simulink model "CAR_CONTROL_SYSTEM"  (R2024b)
settings: Solver=FixedStepAuto  StartTime=0.0  StopTime=inf  FixedStep=1e-3  RelTol=1e-3  EnableMultiTasking=on
model workspace (MAT data in the model file):
  SL_ROS_VariableLengthArrays_MaxSizes : object (value not decoded)
undefined symbols (not defined in the file or in its folder): angular, CIRCUIT, CLTF_DAMP, CLTF_FREQ, CLTF_GAIN, CONTROL, CONTROL_INI, DiscIntNeverNeededParam, dspblkCoreblockFVToolHelper, gcbh, INPUT, linear, MCP3201, MD25, MODEL, MODEL_INI, mpcstate, MPU60X0, MPU9250, MSG, NAV_MPC_CONTROL, OUTPUT, SAMPLING_TIME, SYSID_INPUT, VL6180X
libraries: raspberrypiCommlib x153, simulink x85, raspberrypiNetworklib x8, embedlinuxBasiclib x6, ctrlSharedLib x2, ros2lib x2, mpclib x1, vrlib x1, sldrtlib x1
(part 14 of 16)

== matlab function CAR_CONTROL_SYSTEM/SIMULATION/CAR MODEL  ==
  settings: updateMethod=DISCRETE  sampleTime=MODEL_INI.PARAM.SIM_SAMPLING_TIME
  data: STATE input; MODEL_IN input; STATE_DERIVATIVE output; MODEL output Bus: MODEL_Bus
function [STATE_DERIVATIVE,MODEL] = CAR_MODEL(STATE,MODEL_IN)
%% COPY MODEL_BUS
MODEL = MODEL_IN;

%% Reference frames
% Fixed or earth reference frame
% X,e1I - North
% Y,e2I - East
% Z,e3I - Down
% Body reference frame with origin in the center of mass
% Xb,e1B - forward axis
% Yb,e2B - right axis
% Zb,e3B - downward axis

persistent initialize TIMER
if isempty(initialize)
    TIMER = 0;
    initialize = 1;
end

%--------------------------------------------------------------
% MOTOR PARAMETERS
%--------------------------------------------------------------
% Rotor resistance (ohm)
Rm = MODEL.PARAM.MOTOR_RESISTANCE;
% Motor back-emf constant (V/rad*s)
Ke = MODEL.PARAM.MOTOR_BEMF_CONSTANT;
% Torque constant (N.m/A)
Kt = MODEL.PARAM.MOTOR_TORQUE_CONSTANT;
% Motor static torque (N. m) eje motor
Trmax = MODEL.PARAM.MOTOR_STATIC_TORQUE; 
% Viscous friction coefficient in the motor axis (N.m.s/rad)
Dm = MODEL.PARAM.MOTOR_VISCOUS_FRICTION_COEFF;
% Motor + wheel inertia in the motor axis (kg.m^2)
Im = MODEL.PARAM.MOTOR_INERTIA;
% Motor gear ratio
n1 = MODEL.PARAM.MOTOR_GEAR_RATIO;
% Converter voltage drop (V)
vc_drop = MODEL.PARAM.MOTOR_VOLT_DROP_COM;
vd_drop = MODEL.PARAM.MOTOR_VOLT_DROP_DIF;

%--------------------------------------------------------------
% CAR PARAMETERS
%--------------------------------------------------------------
% Body mass without wheels (kg)
M = MODEL.PARAM.BODY_MASS; 
% Wheel mass including the rotor (kg)
m = MODEL.PARAM.WHEEL_MASS;
% Body inertia in x-axis (kg.m^2)
Ix = MODEL.PARAM.BODY_INERTIA_X;
% Body inertia in y-axis (pitch) (kg.m^2)
Iy = MODEL.PARAM.BODY_INERTIA_Y;
% Body inertia in z-axis (kg.m^2)
Iz = MODEL.PARAM.BODY_INERTIA_Z;
% Viscous friction coefficient in x-axis (N.m.s/rad)
Dx = MODEL.PARAM.BODY_VISCOUS_FRICTION_COEFF_X;
% Viscous friction coefficient in z-axis (N.m.s/rad)
Dz = MODEL.PARAM.BODY_VISCOUS_FRICTION_COEFF_Z;
% Center of gravity distance from the wheel axis (m)
h = MODEL.PARAM.BODY_DISTANCE;
% Wheel radius (m)
R = MODEL.PARAM.WHEEL_RADIUS;
% Distance between wheels (m)
W = MODEL.PARAM.WHEEL_DISTANCE;
% Wheel gear ratio 
n2 = MODEL.PARAM.WHEEL_GEAR_RATIO; 

%--------------------------------------------------------------
% OTHER PARAMETERS
%--------------------------------------------------------------
% Gravity (m/s^2)
g = MODEL.PARAM.GRAVITY;
% Vehicle mode: / 0. CAR / 1. SELF-BALANCING VEHICLE
vmode = MODEL.PARAM.VEHICLE_MODE;
% Yaw and range sensor parameters
if vmode == 0 % CAR
    Iyaw = Iz;
    Dyaw = Dz;
    if MODEL.PARAM.WALL_FOLLOWER_MODE
        xA = MODEL.PARAM.LIDAR_2D_XA;
        yA = MODEL.PARAM.LIDAR_2D_YA;        
    else
        xA = MODEL.PARAM.RANGE_XA;
        yA = MODEL.PARAM.RANGE_YA;
    end
else % SELF-BALANCING VEHICLE
    Iyaw = Ix;
    Dyaw = Dx;
    xA = MODEL.PARAM.RANGE_ZA;
    yA = MODEL.PARAM.RANGE_YA;  
end

%--------------------------------------------------------------
% STATE VARIABLES
%--------------------------------------------------------------
% Forward velocity (m/s)
vc = STATE(1);
% Yaw rate
dShi = STATE(2);
% Yaw angle
Shi = STATE(3);
% Position in earth x-axis (m)
x = STATE(4);
% Position in earth y-axis (m)
y = STATE(5);
% Wall follower mode
if (MODEL.PARAM.CONTROL_MODE == 4) || (MODEL.PARAM.CONTROL_MODE == 5)
    % Wall distance (m)
    d_wall = STATE(6);
    % Wall angle (rad)
    Shi_wall = STATE(7);
else
    d_wall = 0;
    Shi_wall = 0;
end
% Pitch rate (rad/s)
dTheta = STATE(8);
% Pitch angle (rad)
Theta = STATE(9);
if abs(Theta)>=pi/2
    dTheta = 0;
end

%--------------------------------------------------------------
% INPUT VARIABLES
%--------------------------------------------------------------
% Motor voltages (V)
ul = MODEL.INPUT.MOTOR_VOLT(1);
ur = MODEL.INPUT.MOTOR_VOLT(2);
% Wall rotation (rad/s)
w_wall = MODEL.INPUT.WALL_RATE;

%%%%%%%%%%%%%%%%%%%%%%%%%%%%%%%%%%%%%%%%%%%%%%%%%%%%%%%%%%%%%%%%%%%%%%%%%%%
% STATE EQUATIONS
%%%%%%%%%%%%%%%%%%%%%%%%%%%%%%%%%%%%%%%%%%%%%%%%%%%%%%%%%%%%%%%%%%%%%%%%%%%
%--------------------------------------------------------------
% Common  motor voltage (V)
uc = (ul+ur)/2;
% Differential motor voltage (V)
ud = (ul-ur)/2;
%--------------------------------------------------------------
% Differential velocity of the wheels (m/s)
vd = W/2*dShi;
% (wml-wmr)/2/n2*R/W
% Common angular rate of the wheels (rad/s)
wc = vc/R;
% Differential angular rate of the wheels (rad/s)
wd = vd/R;
%--------------------------------------------------------------
% Common angular rate of the motors (rad/s)
wmc = n2*wc + dTheta/n1;
% Differential angular rate of the motors (rad/s)
wmd = n2*wd;
%--------------------------------------------------------------
% Motor rate 
wml = wmc + wmd;
wmr = wmc - wmd;
% wmc = (wmr+wml)/2;
% wmd = (wml-wmr)/2
%--------------------------------------------------------------
% Motor equations
el = Ke*wml;
er = Ke*wmr;
vl_drop = sign(ul-el)*(vc_drop+vd_drop);
vr_drop = sign(ur-er)*(vc_drop-vd_drop);
if abs(ul-el)<vl_drop
    vl_drop = 0;    
end
if abs(ur-er)<vr_drop
    vr_drop = 0;
end
% Currents
il = (ul-vl_drop-el)/Rm;
ir = (ur-vr_drop-er)/Rm;
% ic = (il+ir)/2;
% id = (il-ir)/2;
% dil = (ul - el - Rm*il)/Lm;
% dir = (ur - er - Rm*ir)/Lm;
% Motor torques
Tml = Kt*il;
Tmr = Kt*ir;
Tmc = (Tml+Tmr)/2;
Tmd = (Tml-Tmr)/2;
%--------------------------------------------------------------
% Static friction torques
Trl_lim = Tml*(abs(Tml)<Trmax) - Trmax*(Tml<=-Trmax) + Trmax*(Tml>=Trmax);
Trl = Trl_lim*(abs(wml)==0) + Trmax*sign(wml)*(abs(wml)>0);
Trr_lim = Tmr*(abs(Tmr)<Trmax) - Trmax*(Tmr<=-Trmax) + Trmax*(Tmr>=Trmax);
Trr = Trr_lim*(abs(wmr)==0) + Trmax*sign(wmr)*(abs(wmr)>0);
Trc = (Trl+Trr)/2;
Trd = (Trl-Trr)/2;
%--------------------------------------------------------------
% Viscous friction torques
Tdl = Dm*wml;
Tdr = Dm*wmr;
Tdc = (Tdr+Tdl)/2;
Tdd = (Tdl-Tdr)/2;
%--------------------------------------------------------------
% Total motor torque
% Tl = Tml - Tdl - Trl - Frl*R/n2;
% Tr = Tmr - Tdr - Trr - Frr*R/n2;
%--------------------------------------------------------------
% Motor angular accelerations
% dwml = Tl/Im = (Tml-Tdl-Trl-Frl*R/n2)/Im
% dwmr = Tr/Im = (Tmr-Tdr-Trr-Frr*R/n2)/Im
%--------------------------------------------------------------
% Friction body forces
% Frl = n2/R*(Tml-Tdl-Trl-Im*dwml)
% Frr = n2/R*(Tmr-Tdr-Trr-Im*dwmr)
%--------------------------------------------------------------
if vmode == 0
    %--------------------------------------------------------------
    % Translation equation in x-axis (CAR)
    % Frl + Frr = (M+2*m)*dvc
    % 2*n2/R*(Tmc-Tdc-Trc) = (M+2*m+2*(n2/R)^2*Im)*dvc
    %---------------------------------------------------------    %--------------------------------------------------------------
    % Computation of dvc (CAR)
    dvc = 2*n2/R*(Tmc-Tdc-Trc)/(M+2*m+2*(n2/R)^2*Im);
    d2Theta = 0;
    % (M+2*m+2*(n2/R)^2*Im)*dvc + 2*n2^2/R^2*(Dm+Kt*Ke/Rm)*vc = 2*n2*Kt/R/Rm*uc
    % Tv*dvc + vc = Kv*uc
    % Kv = 2*n2*Kt/R/Rm/(2*(n2/R)^2*(Dm+Kt*Ke/Rm))
    % Tv = (M+2*m+2*(n2/R)^2*Im)/(2*(n2/R)^2*(Dm+Kt*Ke/Rm))
    %--------------------------------------------------------------
else
    %--------------------------------------------------------------
    % Translation equation in x-axis (c)
    % Frl + Frr = (M+2*m)*dvc  - M*h*cos(Theta)*d2Theta + M*h*sin(Theta)*dTheta^2
    % 2*n2/R*(Tmc-Tdc-Trc) - M*h*sin(Theta)*dTheta^2 =
    %    = (M+2*m+2*(n2/R)^2*Im)*dvc  - (M*h*cos(Theta)-2*n2/n1/R*Im)*d2Theta
    %--------------------------------------------------------------
    % Chassis reaction force Nx (SELF-BALANCING VEHICLE)
    % Nx - M*g*sin(Theta) = M*cos(Theta)*dvc - M*h*d2Theta
    % h*Nx + 2*Tc = Iy*d2Theta (2/30*Tc is ignored)
    % Nx = M*cos(Theta)*dvc - M*h*d2Theta + M*g*sin(Theta)
    % M*g*h*sin(Theta) + M*h*cos(Theta)*dvc - M*h^2*d2Theta + 2*Tc = Iy*d2Theta
    % 2*Tc + M*g*h*sin(Theta) = -M*h*cos(Theta)*dvc + (Iy+M*h^2)*d2Theta
    % M*g*h*sin(Theta) = -(M*h*cos(Theta)+2/R*Im)*dvc + (Iy+M*h^2-2*Im/n1^2)*d2Theta
    %--------------------------------------------------------------
    % Computation of dvc and d2Theta (SELF-BALANCING VEHICLE)
    matA = [       M+2*m+2*(n2/R)^2*Im      -(M*h*cos(Theta)-2*n2/n1/R*Im)
             -(M*h*cos(Theta)+2/R*Im)        Iy+M*h^2-2*Im/n1^2      ];
    matB = [   2*n2/R*(Tmc-Tdc-Trc)-M*h*dTheta^2*sin(Theta)
                               M*g*h*sin(Theta) ];
    aux = matA\matB;
    dvc = aux(1);
    d2Theta = aux(2);
    %--------------------------------------------------------------
end
%--------------------------------------------------------------
% Rotation equation in yaw-axis
% Frl - Frr = 2*n2/R*(Tmd-Tdd-Trd-Im*dwmd)
% Torque in yaw-axis (earth reference-frame)
% Tz = (Frl-Frr)*W/2 - Dyaw*dShi
% Iyaw*d2Shi = W/2*(Frl-Frr) - Dyaw*dShi
% Iyaw*d2Shi = n2*W/R*(Tmd-Tdd-Trd-Im*dwmd) - Dyaw*dShi
% wmd = n2*wd = n2/R*vd = n2*W/2/R*dShi
% dwmd = W/R/2*d2Shi
% Iyaw*d2Shi = n2*W/R*(Tmd-Tdd-Trd-Im*n2*W/R/2*d2Shi) - Dyaw*dShi
% (Iyaw+(n2*W/R)^2/2*Im)*d2Shi = n2*W/R*(Tmd-Tdd-Trd) - Dyaw*dShi
d2Shi = 1/(Iyaw+(n2*W/R)^2/2*Im)*(n2*W/R*(Tmd-Tdd-Trd) - Dyaw*dShi);
% (Iyaw+(n2*W/R)^2/2*Im)*d2Shi + Dyaw*dShi + n2*W/R*Tdd  = n2*W/R/Rm*Kt*(ud-ed)
% (Iz+n2*(W/R)^2/2*Im)*d2Shi + Dz*dShi + n2^2/R^2*W^2/2*Dm*dShi + n2^2/R^2*W^2/2*Kt*Ke/Rm*dShi = n2*W/R/Rm*Kt*ud
% Kw = n2/R*W*Kt/Rm/(Dyaw+n2^2/R^2*W^2/2*(Dm+Kt*Ke/Rm))
% Tw = (Iyaw+(n2*W/R)^2/2*Im)/(Dyaw+n2^2/R^2*W^2/2*(Dm+Kt*Ke/Rm))
%---------------------------------------------------------
% Earth velocity
vx = vc*cos(Shi);
vy = vc*sin(Shi);
vz = 0;
vxyz = [vx vy vz]';
dvx = dvc*cos(Shi) - vc*sin(Shi)*dShi;
dvy = dvc*sin(Shi) + vc*cos(Shi)*dShi;
dvz = 0;
dvxyz = [dvx dvy dvz]';
%--------------------------------------------------------------
% Wall distance derivative
dd_wall = 0;
dShi_wall = 0;
% Wall follower model
if (MODEL.PARAM.CONTROL_MODE == 4) || (MODEL.PARAM.CONTROL_MODE == 5)
    dShi_wall = dShi - w_wall; 
    dd_wall = -(vc-dShi_wall*yA)*sin(Shi_wall) - dShi_wall*xA*cos(Shi_wall);
end
if vmode && TIMER<1
    dvc = 0; d2Shi = 0; dShi = 0; vx = 0; vy = 0; dd_wall = 0; 
    dShi_wall = 0; d2Theta = 0; dTheta = 0; dvxyz = zeros(3,1);
    TIMER = TIMER + MODEL.PARAM.SIM_SAMPLING_TIME;
end

%%%%%%%%%%%%%%%%%%%%%%%%%%%%%%%%%%%%%%%%%%%%%%%%%%%%%%%%%%%%%%%%%%%%%%%%%%%
STATE_DERIVATIVE = [dvc ; d2Shi ; dShi ; vx ; vy ; dd_wall ; dShi_wall ; ...
                    d2Theta ; dTheta];
%%%%%%%%%%%%%%%%%%%%%%%%%%%%%%%%%%%%%%%%%%%%%%%%%%%%%%%%%%%%%%%%%%%%%%%%%%%

%%%%%%%%%%%%%%%%%%%%%%%%%%%%%%%%%%%%%%%%%%%%%%%%%%%%%%%%%%%%%%%%%%%%%%%%%%%
% OUTPUT BUS
%%%%%%%%%%%%%%%%%%%%%%%%%%%%%%%%%%%%%%%%%%%%%%%%%%%%%%%%%%%%%%%%%%%%%%%%%%%
% COMPUTATION OF EULER ANGLES, RATES & MATRICES 
if vmode == 0 % CAR
    % Roll angle (rad)
    Phi_car = 0;
    % Roll rate (rad/s)
    dPhi_car = 0;
    % Roll acceleration (rad/s^2)
    d2Phi_car = 0;
    % Pitch angle (rad)
    Theta_car = Theta;
    % Pitch rate (rad/s)
    dTheta_car = dTheta;
    % Pitch acceleration (rad/s^2)
    d2Theta_car = d2Theta;    
    % Yaw angle (rad)
    Shi_car = Shi;
    % Yaw rate (rad/s)
    dShi_car = dShi;
    % Yaw acceleration (rad/s^2)
    d2Shi_car = d2Shi;    
else % SELF-BALANCING VEHICLE
    % Roll angle (rad)
    Phi_car = -Shi;
    % Roll rate (rad/s)
    dPhi_car = -dShi;
    % Roll acceleration (rad/s^2)
    d2Phi_car = -d2Shi;
    % Pitch angle (rad)
    Theta_car = Theta+pi/2-MODEL.PARAM.IMU_PITCH_OFFSET;
    % Pitch rate (rad/s)
    dTheta_car = dTheta;
    % Pitch acceleration (rad/s^2)
    d2Theta_car = d2Theta; 
    % Yaw angle (rad)
    Shi_car = 0;
    % Yaw rate (rad/s)
    dShi_car = 0;
    % Yaw acceleration (rad/s^2)
    d2Shi_car = 0;    
end
MODEL.OUTPUT.EULER_ANG = [Phi_car ; Theta_car ; Shi_car];
MODEL.OUTPUT.EULER_RATE = [dPhi_car ; dTheta_car ; dShi_car];
MODEL.OUTPUT.EULER_RATE_DER = [d2Phi_car ; d2Theta_car ; d2Shi_car];
MODEL.OUTPUT.matDCM_BE = ...
 [ cos(Theta_car)*cos(Shi_car) sin(Phi_car)*sin(Theta_car)*cos(Shi_car)-cos(Phi_car)*sin(Shi_car)  cos(Phi_car)*sin(Theta_car)*cos(Shi_car)+sin(Phi_car)*sin(Shi_car)
   sin(Shi_car)*cos(Theta_car) sin(Phi_car)*sin(Theta_car)*sin(Shi_car)+cos(Phi_car)*cos(Shi_car)  cos(Phi_car)*sin(Theta_car)*sin(Shi_car)-sin(Phi_car)*cos(Shi_car)
  -sin(Theta_car)          sin(Phi_car)*cos(Theta_car)                             cos(Phi_car)*cos(Theta_car)                           ];
MODEL.OUTPUT.matEULER = [ 1     0         -sin(Theta_car)
                          0  cos(Phi_car) sin(Phi_car)*cos(Theta_car)
                          0 -sin(Phi_car) cos(Phi_car)*cos(Theta_car) ];
% matEuler = [ 1     0         -sin(Theta)
%              0  cos(Phi) sin(Phi)*cos(Theta)
%              0 -sin(Phi) cos(Phi)*cos(Theta) ]
MODEL.OUTPUT.matEULER_DER = [ 0          0                         -cos(Theta_car)*dTheta_car
                              0 -sin(Phi_car)*dPhi_car   cos(Phi_car)*cos(Theta_car)*dPhi_car-sin(Phi_car)*sin(Theta_car)*dTheta_car
                              0 -cos(Phi_car)*dPhi_car  -sin(Phi_car)*cos(Theta_car)*dPhi_car-cos(Phi_car)*sin(Theta_car)*dTheta_car ];
% wxyz = matEuler*dEuler;
MODEL.OUTPUT.BODY_RATE = MODEL.OUTPUT.matEULER*MODEL.OUTPUT.EULER_RATE;
% dwxyz = matEuler_der*dEuler + matEuler*d2Euler
MODEL.OUTPUT.BODY_RATE_DER = MODEL.OUTPUT.matEULER*MODEL.OUTPUT.EULER_RATE_DER + ...
                             MODEL.OUTPUT.matEULER_DER*MODEL.OUTPUT.EULER_RATE;
MODEL.OUTPUT.EARTH_VEL = vxyz;
MODEL.OUTPUT.EARTH_POS = [x ; y ; 0];
MODEL.OUTPUT.EARTH_VEL_DER = dvxyz;
MODEL.OUTPUT.BODY_VEL_DER = MODEL.OUTPUT.matDCM_BE'*dvxyz;
MODEL.OUTPUT.FORWARD_VEL = vc;
MODEL.OUTPUT.PITCH_ANG = Theta;
MODEL.OUTPUT.YAW_ANG = Shi;
MODEL.OUTPUT.PITCH_RATE = dTheta;
MODEL.OUTPUT.YAW_RATE = dShi;
MODEL.OUTPUT.MOTOR_VOLT_CD = [uc ; ud];
MODEL.OUTPUT.MOTOR_CURRENT = [il ; ir];
MODEL.OUTPUT.MOTOR_RATE = [wml ; wmr];
MODEL.OUTPUT.WHEEL_RATE = MODEL.OUTPUT.MOTOR_RATE/n2;
MODEL.OUTPUT.WALL_DIST = d_wall;
MODEL.OUTPUT.WALL_ANG = Shi_wall;

return

== matlab function CAR_CONTROL_SYSTEM/HARDWARE/SENSORS/IMU MPU60X0_SPI/READ FIFO/FIFO_PROCESSING ==
  data: CONTROL_IN input Bus: CONTROL_Bus; FIFO_DATA input; CONTROL_OUT output Bus: CONTROL_Bus; FIFO_LENGTH input; RAW_GYRO_MEAN_OUT output; RAW_ACCEL_MEAN_OUT output; ACCEL_SSF input; GYRO_SSF input; ACCEL_FIFO output; GYRO_FIFO output
function [CONTROL_OUT,RAW_GYRO_MEAN_OUT,RAW_ACCEL_MEAN_OUT,ACCEL_FIFO,GYRO_FIFO] = FIFO_PROCESSING(CONTROL_IN,FIFO_DATA,FIFO_LENGTH,ACCEL_SSF,GYRO_SSF)

%% INITIALIZATION
FIFO_DATA = FIFO_DATA(:);
AUX = single(zeros(3,FIFO_LENGTH));
GRAVITY = CONTROL_IN.PARAM.GRAVITY;
GYRO_FIFO = zeros(30,1,'single');
ACCEL_FIFO = zeros(30,1,'single');

%% GYROSCOPE
for nn = 1:FIFO_LENGTH
    ii = 2*nn;
    AUX(:,nn) = single(FIFO_DATA(3*(ii-1)+1:3*ii));
end
RAW_GYRO_MEAN = sum(AUX,2)/single(FIFO_LENGTH);
RAW_GYRO = AUX(:,end);
GYRO_FIFO(1:30) = [AUX(1,:) AUX(2,:) AUX(3,:)]'/GYRO_SSF*pi/180;


%% ACCELEROMETER
for nn = 1:FIFO_LENGTH
    ii = 2*nn-1;
    AUX(:,nn) = single(FIFO_DATA(3*(ii-1)+1:3*ii));
end
RAW_ACCEL_MEAN = sum(AUX,2)/single(FIFO_LENGTH);
RAW_ACCEL = AUX(:,end);
ACCEL_FIFO(1:30) = [AUX(1,:) AUX(2,:) AUX(3,:)]'/ACCEL_SSF*GRAVITY;

%% SENSOR BUS UPDATE
CONTROL_OUT = CONTROL_IN;
CONTROL_OUT.INPUT.IMU.RAW_GYRO = int16(RAW_GYRO);
CONTROL_OUT.INPUT.IMU.RAW_ACCEL = int16(RAW_ACCEL);
RAW_GYRO_MEAN_OUT = int16(RAW_GYRO_MEAN);
RAW_ACCEL_MEAN_OUT = int16(RAW_ACCEL_MEAN);

== matlab function CAR_CONTROL_SYSTEM/HARDWARE/SENSORS/IMU MPU60X0_SPI/READ TEMP/IMU SCALING ==
  data: CONTROL_IN input; CONTROL_OUT output Bus: SENSOR_Bus; TEMP_SSF input; TEMP_OFFS input
function CONTROL_OUT = IMU_SCALING(CONTROL_IN,TEMP_SSF,TEMP_OFFS)

%% INPUT
CONTROL_OUT = CONTROL_IN;
RAW_TEMP = CONTROL_OUT.IMU.TEMP;

%% TEMP SCALING
SCALED_TEMP = int16(100*(single(RAW_TEMP)/TEMP_SSF + TEMP_OFFS)); % ºC/100
TEMP = single(100*SCALED_TEMP);

%% IMU BUS UPDATE
CONTROL_OUT.INPUT.IMU.SCALED_TEMP = SCALED_TEMP;
CONTROL_OUT.INPUT.IMU.TEMP = TEMP;

== matlab function CAR_CONTROL_SYSTEM/NAVIGATION/NAVIGATION TARGETS/TRAJECTORY PLANNER (POLYNOMIAL IN Vx & Vy) ==
  data: CONTROL_IN input Bus: CONTROL_Bus; CONTROL output Bus: CONTROL_Bus
function CONTROL = MPC_TARGET_UPDATE(CONTROL_IN)

%--------------------------------------------------------------
% COPY CONTROL BUS
%--------------------------------------------------------------
CONTROL = CONTROL_IN;

%--------------------------------------------------------------
% DISABLING TARGET UPDATE
%--------------------------------------------------------------
% CONTROL_STATUS
% / 0. INITIALIZATION     / 1. ESTIMATION    / 2. ACTIVE CONTROL
if CONTROL.STATE.CONTROL_STATUS < 2  % INITIALIZATION    
    return
end

%--------------------------------------------------------------
% TIME MANAGEMENT
%--------------------------------------------------------------
% Sampling time 
ts = CONTROL.PARAM.SAMPLING_TIME;
% Trajectory update time 
tc = 10*ts;
persistent initialize TIMER
if isempty(initialize)
    TIMER = 0;
    initialize = 1;
end
TIMER = TIMER + ts;
if TIMER > tc-ts/2
    TIMER = 0;
    return
end

%--------------------------------------------------------------
% PARAMETERS
%--------------------------------------------------------------
% Maximun velocity magnitude 
VEL_MAG_MAX = CONTROL.PARAM.VEL_MAG_MAX;
% Prediction horizon (<= prediction horizon in mpcDesigner)
P = 20;
% Circular outline radius
% WP_R = CONTROL.PARAM.WP_R;

%--------------------------------------------------------------
% MEASUREMENTS AND STATE
%--------------------------------------------------------------
VEL_MAG = CONTROL.INPUT.FORWARD_VEL;
VEL_ANG = CONTROL.INPUT.YAW_ANG;
VEL_X = CONTROL.INPUT.EARTH_VEL(1);
VEL_Y = CONTROL.INPUT.EARTH_VEL(2);
POS_XY = CONTROL.INPUT.EARTH_POS(1:2);
WP_XY = CONTROL.TARGET.MISSION_WAYPOINTS(1:CONTROL.TARGET.MISSION_NUM_WAYPOINTS,2:3)';
NEXT_WP = CONTROL.TARGET.MISSION_COUNT;
M = CONTROL.PARAM.NAV_MPC.PRED_HRZ;
if NEXT_WP == size(WP_XY,2)
    CONTROL.TARGET.NAV_REF_LC(1) = 0;
    CONTROL.TARGET.NAV_REF(1) = 0;
    CONTROL.TARGET.NAV_REF_MPC(1:M,1) = zeros(M,1);
    CONTROL.TARGET.VEL_XY_REF(1) = 0;
    CONTROL.TARGET.VEL_XY_REF(2) = 0;
    CONTROL.TARGET.FORWARD_VEL_REF = 0;
end

%--------------------------------------------------------------
% TRAJECTORY PLANNING
%--------------------------------------------------------------
% x(t) = sum(ai*t^i) i=0...N
% y(t) = sum(bi*t^i) i=0...N
% dx(t)/dt = vx(t) = sum(i*ai*t^(i-1)) i=0...N
% dy(t)/dt = vy(t) = sum(i*bi*t^(i-1)) i=0...N
% Position and distance data
pos_x = [POS_XY(1) WP_XY(1,NEXT_WP:end)]';
pos_y = [POS_XY(2) WP_XY(2,NEXT_WP:end)]'; 
d = abs(diff(pos_x) + 1j*diff(pos_y));
% Delete duplicated points (distance = 0)
ind = find(d>0);
pos_x = [pos_x(ind) ; pos_x(end)];
pos_y = [pos_y(ind) ; pos_y(end)];
d = abs(diff(pos_x) + 1j*diff(pos_y));
% Polynomial parameters
Np = min([4 length(pos_x)+1]);
% Polynomial order
N = Np-1;
% Parameter initialization
a = zeros(Np,1);
b = zeros(Np,1);
a(1) = pos_x(1);
b(1) = pos_y(1);
a(2) = VEL_X;
b(2) = VEL_Y;
% Time vector for target
t_tgt = (1:P)'*tc;
VEL_MAG_TARGET = zeros(P,1);
VEL_ANG_TARGET = zeros(P,1);
% Time matrix for velocity target computation
matTp = zeros(P,N+1);
matTv = zeros(P,N);
for nn = 1:N+1
    matTp(:,nn) = t_tgt.^(nn-1);
end
for nn = 1:N
    matTv(:,nn) = nn*t_tgt.^(nn-1);
end
flag_vel_max = true;
k = 1;
while flag_vel_max
    % Reaching time for the next waypoints
    t = cumsum([0 ; k*sqrt(2)*d(1:N-1)/VEL_MAG_MAX]);    
    % Polynomial coefficient estimation 
    % matBx = matA*a(3:Np);  
    % matBy = matA*b(3:Np)
    matA = zeros(Np-2);
    for nn = 1:Np-2
        matA(:,nn) = t(2:end).^(nn+1);
    end
    matBx = pos_x(2:Np-1) - a(2)*t(2:end) - a(1);
    matBy = pos_y(2:Np-1) - b(2)*t(2:end) - b(1);
    inv_matA = inv(matA);
    a(3:end) = inv_matA*matBx;
    b(3:end) = inv_matA*matBy;
    % Position target calculation
    px_tgt = matTp*a;
    py_tgt = matTp*b; 
    % Magnitude and angle velocity targets calculation
    vx_tgt = matTv*a(2:end);
    vy_tgt = matTv*b(2:end); 
    v_tgt = vx_tgt + 1j*vy_tgt;
    VEL_MAG_TARGET = abs(v_tgt);
    VEL_ANG_TARGET = angle(v_tgt)*(VEL_MAG_TARGET(1)>=0.005) + ...
                    VEL_ANG*ones(size(VEL_ANG_TARGET))*(VEL_MAG_TARGET(1)<0.005);
    % Decreasing velocity factor
    k = k*max(VEL_MAG_TARGET)/VEL_MAG_MAX;
    % Maximun velocity verification
    if (max(VEL_MAG_TARGET)/VEL_MAG_MAX)<=1.01
        flag_vel_max = false;
    end
end

%--------------------------------------------------------------
% UNWRAPPING
%--------------------------------------------------------------
aux1 = VEL_ANG_TARGET(1);
aux2 = VEL_ANG;
INC_VEL_ANG_TARGET = zeros(21,1);
INC_VEL_ANG_TARGET(1) = aux1-aux2;
for nn=1:10
    INC_VEL_ANG_TARGET(2*nn:2*nn+1) = [aux1-aux2-2*nn*pi ; aux1-aux2+2*nn*pi];
end
[~,ind] = min(abs(INC_VEL_ANG_TARGET));
VEL_ANG_TARGET(1) = aux2 + INC_VEL_ANG_TARGET(ind);
for nn = 2:P
    INC_VEL_ANG_TARGET = [VEL_ANG_TARGET(nn)-VEL_ANG_TARGET(nn-1)
                          VEL_ANG_TARGET(nn)-VEL_ANG_TARGET(nn-1)-2*pi
                          VEL_ANG_TARGET(nn)-VEL_ANG_TARGET(nn-1)+2*pi];
    [~,ind] = min(abs(INC_VEL_ANG_TARGET));
    VEL_ANG_TARGET(nn) = VEL_ANG_TARGET(nn-1) + INC_VEL_ANG_TARGET(ind);
end

%--------------------------------------------------------------
% CONTROL BUS UPDATE
%--------------------------------------------------------------
CONTROL.TARGET.NAV_REF_LC(1) = VEL_MAG_TARGET(1);
CONTROL.TARGET.NAV_REF_LC(2) = VEL_ANG_TARGET(1);
if M<=P
    CONTROL.TARGET.NAV_REF_MPC(1:M,1) = VEL_MAG_TARGET(1:M);
    CONTROL.TARGET.NAV_REF_MPC(1:M,2) = VEL_ANG_TARGET(1:M);
else
    CONTROL.TARGET.NAV_REF_MPC(1:M,1) = [VEL_MAG_TARGET(1:P); VEL_MAG_TARGET(end)*ones(M-P,1)];
    CONTROL.TARGET.NAV_REF_MPC(1:M,2) = [VEL_ANG_TARGET(1:P); VEL_ANG_TARGET(end)*ones(M-P,1)];
end
VEL_XY = VEL_MAG_TARGET.*exp(1j*VEL_ANG_TARGET);
CONTROL.TARGET.VEL_XY_REF(1) = real(VEL_XY(1));
CONTROL.TARGET.VEL_XY_REF(2) = imag(VEL_XY(1));
CONTROL.TARGET.NAV_REF = [VEL_MAG_TARGET(1) ; VEL_ANG_TARGET(1)];

return

== matlab function CAR_CONTROL_SYSTEM/CONTROL/LOCAL TARGETS/NAVIGATION TARGETS/PATH PLANNER ==
  data: CONTROL_IN input Bus: CONTROL_Bus; CONTROL output Bus: CONTROL_Bus
function CONTROL = MPC_TARGET_UPDATE(CONTROL_IN)

%--------------------------------------------------------------
% COPY CONTROL BUS
%--------------------------------------------------------------
CONTROL = CONTROL_IN;

%--------------------------------------------------------------
% DISABLING TARGET UPDATE
%--------------------------------------------------------------
% CONTROL_STATUS
% / 0. INITIALIZATION     / 1. ESTIMATION    / 2. ACTIVE CONTROL
if CONTROL.STATE.CONTROL_STATUS < 2  % INITIALIZATION    
    return
end

%--------------------------------------------------------------
% TIME MANAGEMENT
%--------------------------------------------------------------
% Sampling time 
ts = CONTROL.PARAM.SAMPLING_TIME;
% Trajectory update time 
tc = 10*ts;
persistent initialize TIMER
if isempty(initialize)
    TIMER = 0;
    initialize = 1;
end
TIMER = TIMER + ts;
if TIMER > tc-ts/2
    TIMER = 0;
    return
end

%--------------------------------------------------------------
% PARAMETERS
%--------------------------------------------------------------
% Maximun velocity magnitude 
VEL_MAG_MAX = CONTROL.PARAM.VEL_MAG_MAX;
% Prediction horizon (<= prediction horizon in mpcDesigner)
P = 20;
% Circular outline radius
% WP_R = CONTROL.PARAM.WP_R;

%**************************************************************************

% Number of waypoints
NUM_WAYPOINTS = CONTROL.TARGET.MISSION_NUM_WAYPOINTS;
% Waypoint list
WP_LIST = CONTROL.TARGET.MISSION_WAYPOINTS(1:NUM_WAYPOINTS,:);
% Next waypoint
NEXT_WP = CONTROL.TARGET.MISSION_COUNT;
% TARGETS
CONTROL.TARGET.NAV_REF = CONTROL.TARGET.NAV_REF_LC;
CONTROL.TARGET.FORWARD_VEL_REF = CONTROL.TARGET.NAV_REF(1);
% Tolerances
WP_R = CONTROL.TARGET.MISSION_WP_RADIUS;
YA_ERR = CONTROL.TARGET.MISSION_YA_ERROR;
% POSITION UPDATE
POS_XY = CONTROL.INPUT.EARTH_POS(1:2);
YAW_ANG = CONTROL.INPUT.YAW_ANG;
POS_INC = (WP_LIST(NEXT_WP,2) - POS_XY(1)) + (WP_LIST(NEXT_WP,3) - POS_XY(2))*1i;
POS_INC_MAG = abs(POS_INC);
if POS_INC_MAG<WP_R
    if WP_LIST(NEXT_WP,1)>TIMER_NAV
        CONTROL.TARGET.FORWARD_VEL_REF = 0;
        CONTROL.TARGET.YAW_ANG_REF = WP_LIST(NEXT_WP,4)*pi/180;
        TIMER_NAV = TIMER_NAV + SAMPLING_TIME;
        if abs(CONTROL.TARGET.YAW_ANG_REF-YAW_ANG)>YA_ERR
            TIMER_NAV = 0;
        end
    else
        TIMER_NAV = 0;
        NEXT_WP = NEXT_WP + uint8(1);
        CONTROL.TARGET.FORWARD_VEL_REF = CONTROL.TARGET.NAV_REF(1);
        CONTROL.TARGET.YAW_ANG_REF = CONTROL.TARGET.NAV_REF(2);
    end
else
    CONTROL.TARGET.FORWARD_VEL_REF = CONTROL.TARGET.NAV_REF(1);
    CONTROL.TARGET.YAW_ANG_REF = CONTROL.TARGET.NAV_REF(2);
end
if NEXT_WP>size(WP_LIST,1)
    NEXT_WP = uint8(size(WP_LIST,1));
end
% CONTROL BUS UPDATE
CONTROL.TARGET.MISSION_COUNT = NEXT_WP;
CONTROL.TARGET.POS_XY_REF = WP_LIST(NEXT_WP,2:3)';
CONTROL.STATE.NEXT_WP = NEXT_WP;

%**************************************************************************            
VEL_XY = VEL_MAG_TARGET.*exp(1j*VEL_ANG_TARGET);
CONTROL.TARGET.VEL_XY_REF(1) = real(VEL_XY(1));
CONTROL.TARGET.VEL_XY_REF(2) = imag(VEL_XY(1));
CONTROL.TARGET.NAV_REF = [VEL_MAG_TARGET(1) ; VEL_ANG_TARGET(1)];

return

== matlab function CAR_CONTROL_SYSTEM/GAZEBO SIMULATION/TCP_BRIDGE/TCP//IP SIM HW/RPI4 CODER ==
  data: CONTROL input; TX_MSG output uint8
function TX_MSG  = RPI4_CODER(CONTROL)
%%%%%%%%%%%%%%%%%%%%%%%%%%%%%%%%%%%%%%%%%%%%%%%%%%%%%%%%%%%%%%%%%%%%%%%%%%%
% MCS MESSAGES
%%%%%%%%%%%%%%%%%%%%%%%%%%%%%%%%%%%%%%%%%%%%%%%%%%%%%%%%%%%%%%%%%%%%%%%%%%%
% WRITE IN THE CONTROL BUS
% RPi3 --> RPi4 (coder)
%       Estado (1B): 1 uint8
%       Comandos tension (16B): 2 double (float64) izquierda y derecha
%             Total: 17B
TX_MSG = zeros(17,1,'uint8');
ii = 1; jj = 1;
TX_MSG(ii-jj+1:ii) = uint8(CONTROL.STATE.CURRENT_STATUS_SYS);
ii = 1 + 1*8; jj = 8;
TX_MSG(ii-jj+1:ii) = typecast(double(CONTROL.OUTPUT.MOTOR_VOLT(1)),'uint8');
ii = 1 + 2*8; jj = 8;
TX_MSG(ii-jj+1:ii) = typecast(double(CONTROL.OUTPUT.MOTOR_VOLT(2)),'uint8');

%%%%%%%%%%%%%%%%%%%%%%%%%%%%%%%%%%%%%%%%%%%%%%%%%%%%%%%%%%%%%%%%%%%%%%%%%%%


return

== matlab function CAR_CONTROL_SYSTEM/GAZEBO SIMULATION/TCP_BRIDGE/TCP//IP SIM HW/RPI4 DECODER ==
  data: CONTROL_IN input; RX_MSG input; CONTROL output Bus: CONTROL_Bus; STATUS input; IMU output; ENCODER output; LATERAL_DIST output
function [CONTROL, IMU, ENCODER, LATERAL_DIST]  = RPI4_DECODER(CONTROL_IN,RX_MSG,STATUS)
% Initialization
CONTROL = CONTROL_IN;
%%%%%%%%%%%%%%%%%%%%%%%%%%%%%%%%%%%%%%%%%%%%%%%%%%%%%%%%%%%%%%%%%%%%%%%%%%%
% MCS MESSAGES
%%%%%%%%%%%%%%%%%%%%%%%%%%%%%%%%%%%%%%%%%%%%%%%%%%%%%%%%%%%%%%%%%%%%%%%%%%%
% Host --> RPi (decoder)
%       Botones (3B): 3 bool (uint8) A, B, C
%       Medidas encoders (8B): 2 double (int32) encoder izquierdo y derecho
%      METER CODIGO PROCESAMIENTO ENCODERS
%      Medidas dist. lateral (8B): 2 single (float32) frontal y trasero
%      METER ANGLE AND DISTANCE COMPUTATION
%      IMU (48B): 3 double (float64) aceleracion y 3 double (float64) giro
%      METER FLITRADO
%      Tension bateria (4B): 1 single (float32)

%       TOTAL: 71B
% WRITE IN THE CONTROL BUS
ENCODER = zeros(2,1);
IMU = zeros(6,1);
LATERAL_DIST = zeros(2,1);

if STATUS==1
    %% VIRTUAL BUTTONS
    ii = 1; jj = 1;
    CONTROL.STATE.BUTTONS(1) = CONTROL.STATE.NAV_BUTTONS(1) || RX_MSG(ii-jj+1:ii);
    ii = 2;
    CONTROL.STATE.BUTTONS(2) = CONTROL.STATE.NAV_BUTTONS(2) || RX_MSG(ii-jj+1:ii);
    ii = 3; 
    CONTROL.STATE.BUTTONS(3) = CONTROL.STATE.NAV_BUTTONS(3) || RX_MSG(ii-jj+1:ii);
    %% ENCODERS
    ii =3 + 4; jj = 4;
    ENCODER(1) = double(typecast(RX_MSG(ii-jj+1:ii),'int32'));
    ii = 3 + 2*4;
    ENCODER(2) = double(typecast(RX_MSG(ii-jj+1:ii),'int32'));
    %% LATERAL DISTANCE SENSORS
    ii = 11 + 4; jj = 4;
    LATERAL_DIST(1) = double(typecast(RX_MSG(ii-jj+1:ii),'single'));
    ii = 11 + 2*4;
    LATERAL_DIST(2) = double(typecast(RX_MSG(ii-jj+1:ii),'single'));
    %% IMU
    ii = 19 + 8; jj = 8;
    IMU(1) = typecast(RX_MSG(ii-jj+1:ii),'double');
    ii = 19 + 2*8;
    IMU(2) = typecast(RX_MSG(ii-jj+1:ii),'double');
    ii = 19 + 3*8;
    IMU(3) = typecast(RX_MSG(ii-jj+1:ii),'double');
    ii = 19 + 4*8;
    IMU(4) = typecast(RX_MSG(ii-jj+1:ii),'double');
    ii = 19 + 5*8;
    IMU(5) = typecast(RX_MSG(ii-jj+1:ii),'double');
    ii = 19 + 6*8;
    IMU(6) = typecast(RX_MSG(ii-jj+1:ii),'double');
    %% BATTERY VOLT
    ii = 67 + 4; jj = 4;
    % CONTROL.INPUT.BATTERY_VOLT = double(typecast(RX_MSG(ii-jj+1:ii),'single'));
end
%%%%%%%%%%%%%%%%%%%%%%%%%%%%%%%%%%%%%%%%%%%%%%%%%%%%%%%%%%%%%%%%%%%%%%%%%%%


return

== matlab function CAR_CONTROL_SYSTEM/CONTROL/ADAPTIVE CONTROL STR/PI DESIGN ==
  data: PARAM input; K_out output; Ti_out output; b_out output; FLAG_ADPT_out output; CONTROL input Bus: CONTROL_Bus
function [K_out,Ti_out,b_out,FLAG_ADPT_out] = PI_DESIGN(PARAM,CONTROL)

%--------------------------------------------------------------
% PERSISTENT VARIABLES
%--------------------------------------------------------------
persistent TIMER K Ti b FLAG_ADPT initialize
if isempty(initialize)
    TIMER = 0;
    K = CONTROL.PARAM.FORWARD_VEL_PID.K;
    Ti = CONTROL.PARAM.FORWARD_VEL_PID.Ti;
    b = CONTROL.PARAM.FORWARD_VEL_PID.b;
    FLAG_ADPT = false;
    initialize = 1;
end

TIMER = TIMER + CONTROL.PARAM.SAMPLING_TIME;
if TIMER < 2
    K_out = K;
    Ti_out = Ti;
    b_out = b;
    FLAG_ADPT_out = FLAG_ADPT; 
    return
else
    TIMER = 0;
end

%% TRANSFER FUNCTION COEFFICIENTS
a1 = -PARAM(1);
a2 = -PARAM(2);
b0 = PARAM(3);

%% SPECIFICATIONS
wn = 10;
seta = 0.7;

%% CONTROL PARAMETERS
tao = a2/(a1-2*a2*seta*wn);
K = (a2*wn^2+2*a2*seta*wn/tao-1)/b0;
Ti = b0*K*tao/a2/wn^2;
b = tao/Ti;
FLAG_ADPT = false;
if K>0 && Ti>0 && tao>0 && b>0
    FLAG_ADPT = true;
end
K_out = K;
Ti_out = Ti;
b_out = b;
FLAG_ADPT_out = FLAG_ADPT;

== matlab function CAR_CONTROL_SYSTEM/GAZEBO SIMULATION/TCP_BRIDGE/TCP//IP SIM HW/Subsystem/GRAVITY ROTATION ==
  data: PITCH_OFFSET input; GRAVITY_VECTOR output; GRAVITY input; VEHICLE_MODE input
function GRAVITY_VECTOR = GRAVITY_ROTATION(PITCH_OFFSET,GRAVITY,VEHICLE_MODE)
if VEHICLE_MODE
    ROTATION_MATRIX = [cos(PITCH_OFFSET) 0 -sin(PITCH_OFFSET) ; 0 1 0 ; sin(PITCH_OFFSET) 0 cos(PITCH_OFFSET)];
    GRAVITY_VECTOR = ROTATION_MATRIX*[GRAVITY ; 0 ; 0];
else
    GRAVITY_VECTOR = [0 ; 0 ; -GRAVITY];
end

== matlab function CAR_CONTROL_SYSTEM/GAZEBO SIMULATION/TCP_BRIDGE/TCP//IP SIM HW/Subsystem/IMU CALIBRATION ==
  data: CONTROL_IN input; ACCEL input; ACCEL_FILT input; ACCEL_MEAN input; ACCEL_MEAN_FILT input; GYRO input; GYRO_FILT input; GYRO_MEAN input; GYRO_MEAN_FILT input; ACCEL_CALIB input; ALFA_CALIB input; ACCEL_OFFS_IN input; GYRO_OFFS_IN input; CONTROL output Bus: CONTROL_Bus; ACCEL_OFFS_OUT output; GYRO_OFFS_OUT output; GRAVITY_VECTOR input
function [CONTROL,ACCEL_OFFS_OUT,GYRO_OFFS_OUT] = IMU_CALIBRATION(CONTROL_IN,...
                       ACCEL,ACCEL_FILT,ACCEL_MEAN,ACCEL_MEAN_FILT,...
                       GYRO,GYRO_FILT,GYRO_MEAN,GYRO_MEAN_FILT,...
                       ACCEL_CALIB,ALFA_CALIB,ACCEL_OFFS_IN,GYRO_OFFS_IN,GRAVITY_VECTOR)
                        
%--------------------------------------------------------------
% COPY CONTROL BUS
%--------------------------------------------------------------
CONTROL = CONTROL_IN;

%--------------------------------------------------------------
% IMU ORIENTATION
%--------------------------------------------------------------
% ACCEL = [0 0 1 ; 1 0 0 ; 0 1 0]*ACCEL;
% GYRO = [0 0 1 ; 1 0 0 ; 0 1 0]*GYRO;
ACCEL_MEAN = [0 0 1 ; 1 0 0 ; 0 1 0]*ACCEL_MEAN;
GYRO_MEAN = [0 0 1 ; 1 0 0 ; 0 1 0]*GYRO_MEAN;
% ACCEL_FILT = [0 0 1 ; 1 0 0 ; 0 1 0]*ACCEL_FILT;
% GYRO_FILT = [0 0 1 ; 1 0 0 ; 0 1 0]*GYRO_FILT;
ACCEL_MEAN_FILT = [0 0 1 ; 1 0 0 ; 0 1 0]*ACCEL_MEAN_FILT;
GYRO_MEAN_FILT = [0 0 1 ; 1 0 0 ; 0 1 0]*GYRO_MEAN_FILT;

%--------------------------------------------------------------
% CALIBRATION 
%--------------------------------------------------------------
if CONTROL.STATE.CURRENT_STATUS_SYS == 1  % CALIBRATION ENABLED
    if ACCEL_CALIB % ACCELEROMETER CALIBRATION ENABLED
        ACCEL_OFFS_OUT = ALFA_CALIB*ACCEL_OFFS_IN + (1-ALFA_CALIB)*(ACCEL_MEAN_FILT-GRAVITY_VECTOR);
    else
        ACCEL_OFFS_OUT = ACCEL_OFFS_IN;
    end
    GYRO_OFFS_OUT  = ALFA_CALIB*GYRO_OFFS_IN  + (1-ALFA_CALIB)*GYRO_MEAN_FILT;
else % END OF CALIBRATION
    ACCEL_OFFS_OUT = ACCEL_OFFS_IN;  
    GYRO_OFFS_OUT  = GYRO_OFFS_IN;
    % ACCEL = ACCEL - ACCEL_OFFS_OUT;
    % GYRO = GYRO - GYRO_OFFS_OUT;
    ACCEL_MEAN = ACCEL_MEAN - ACCEL_OFFS_OUT;
    GYRO_MEAN = GYRO_MEAN - GYRO_OFFS_OUT;
    % ACCEL_FILT = ACCEL_FILT - ACCEL_OFFS_OUT;
    % GYRO_FILT = GYRO_FILT - GYRO_OFFS_OUT;
    ACCEL_MEAN_FILT = ACCEL_MEAN_FILT - ACCEL_OFFS_OUT;
    GYRO_MEAN_FILT = GYRO_MEAN_FILT - GYRO_OFFS_OUT;
end

%--------------------------------------------------------------
% IMU BUS UPDATE
%--------------------------------------------------------------
% CONTROL.INPUT.IMU_ACCEL = ACCEL;
% CONTROL.INPUT.IMU_GYRO = GYRO;
CONTROL.INPUT.IMU_ACCEL_MEAN = ACCEL_MEAN;
CONTROL.INPUT.IMU_GYRO_MEAN = GYRO_MEAN;
% CONTROL.INPUT.IMU_ACCEL_FILT = ACCEL_FILT;
% CONTROL.INPUT.IMU_GYRO_FILT = GYRO_FILT;
CONTROL.INPUT.IMU_ACCEL_MEAN_FILT = ACCEL_MEAN_FILT;
CONTROL.INPUT.IMU_GYRO_MEAN_FILT = GYRO_MEAN_FILT;

return

== matlab function CAR_CONTROL_SYSTEM/GAZEBO SIMULATION/TCP_BRIDGE/TCP//IP SIM HW/READ_ENCODER ==
  data: CONTROL_IN input Bus: CONTROL_Bus; ENCODER input; CONTROL output Bus: CONTROL_Bus
function CONTROL = READ_ENCODER(CONTROL_IN,ENCODER)

%--------------------------------------------------------------
% UPDATE BUS
%--------------------------------------------------------------
CONTROL = CONTROL_IN;

%--------------------------------------------------------------
% STATE
%--------------------------------------------------------------
persistent initialize left_enc_prv right_enc_prv inc_com_ang_prv ...
           inc_dif_ang_prv inc2_com_ang_prv inc2_dif_ang_prv dif_ang ...
           dif_ang_offs left_enc_offs right_enc_offs

if isempty(initialize)
    left_enc_prv = zeros(2,1);
    right_enc_prv = zeros(2,1);
    left_enc_offs = 0;
    right_enc_offs = 0;
    inc_com_ang_prv = zeros(5,1);
    inc_dif_ang_prv = zeros(5,1);
    inc2_com_ang_prv = zeros(5,1);
    inc2_dif_ang_prv = zeros(5,1);
    dif_ang = 0;
    dif_ang_offs = 0;        
    initialize = 1;
end

%--------------------------------------------------------------
% PARAMETERS
%--------------------------------------------------------------
% Wheel gear ratio
WHEEL_GEAR_RATIO = CONTROL.PARAM.WHEEL_GEAR_RATIO;
% Motor gear ratio
MOTOR_GEAR_RATIO = CONTROL.PARAM.MOTOR_GEAR_RATIO;
% Encoder resolution: number of pulses / revolution of main shaft
MOTOR_ENC_RES = CONTROL.PARAM.MOTOR_ENC_RES; 

%--------------------------------------------------------------
% ENCODER READOUT
%--------------------------------------------------------------
right_enc = ENCODER(1);
left_enc = ENCODER(2); 
inc_right_enc = right_enc - right_enc_prv(1);
inc_left_enc = left_enc - left_enc_prv(1);
inc2_right_enc = right_enc - 2*right_enc_prv(1) + right_enc_prv(2);
inc2_left_enc = left_enc - 2*left_enc_prv(1) + left_enc_prv(2);
inc_right_ang = 360/MOTOR_ENC_RES/MOTOR_GEAR_RATIO/WHEEL_GEAR_RATIO*inc_right_enc;
inc_left_ang = 360/MOTOR_ENC_RES/MOTOR_GEAR_RATIO/WHEEL_GEAR_RATIO*inc_left_enc;
inc2_right_ang = 360/MOTOR_ENC_RES/MOTOR_GEAR_RATIO/WHEEL_GEAR_RATIO*inc2_right_enc;
inc2_left_ang = 360/MOTOR_ENC_RES/MOTOR_GEAR_RATIO/WHEEL_GEAR_RATIO*inc2_left_enc;
inc_com_ang = (inc_left_ang + inc_right_ang)/2;
inc_dif_ang = (inc_left_ang - inc_right_ang)/2;
inc2_com_ang = (inc2_left_ang + inc2_right_ang)/2;
inc2_dif_ang = (inc2_left_ang - inc2_right_ang)/2;
% Define first-order incremental encoder threshold 
THR_INC_ENC_DEG = 10; 
% Define second-order incremental encoder threshold 
THR_INC2_ENC_DEG = 1; 
% Check incremental limits
if (abs(inc_right_ang)>THR_INC_ENC_DEG)   || ...
   (abs(inc_left_ang)>THR_INC_ENC_DEG)    || ...
   (abs(inc2_right_ang)>THR_INC2_ENC_DEG) || ...
   (abs(inc2_left_ang)>THR_INC2_ENC_DEG)
    inc2_com_ang = mean(inc2_com_ang_prv);
    inc2_dif_ang = mean(inc2_dif_ang_prv);
    inc_com_ang = mean(inc_com_ang_prv) + inc2_com_ang;
    inc_dif_ang = mean(inc_dif_ang_prv) + inc2_dif_ang;
end
% Update differential angles
dif_ang = dif_ang + inc_dif_ang;
% Update previous values
left_enc_prv(2) = left_enc_prv(1);
right_enc_prv(2) = right_enc_prv(1);
left_enc_prv(1) = left_enc;
right_enc_prv(1) = right_enc;
inc_com_ang_prv = [inc_com_ang ; inc_com_ang_prv(1:end-1)];
inc_dif_ang_prv = [inc_dif_ang ; inc_dif_ang_prv(1:end-1)];
inc2_com_ang_prv = [inc2_com_ang ; inc2_com_ang_prv(1:end-1)];
inc2_dif_ang_prv = [inc2_dif_ang ; inc2_dif_ang_prv(1:end-1)];

%--------------------------------------------------------------
% CALIBRATION 
%--------------------------------------------------------------
ALFA_CALIB = 0.99;
if CONTROL.STATE.CURRENT_STATUS_SYS == 1  % CALIBRATION ENABLED
    dif_ang_offs  = ALFA_CALIB*dif_ang_offs  + (1-ALFA_CALIB)*dif_ang;
    left_enc_offs = ALFA_CALIB*left_enc_offs  + (1-ALFA_CALIB)*left_enc;
    right_enc_offs = ALFA_CALIB*right_enc_offs  + (1-ALFA_CALIB)*right_enc;
elseif CONTROL.STATE.CURRENT_STATUS_SYS == 0
    return
else
end 

%--------------------------------------------------------------
% ENCODER ANGLES
%--------------------------------------------------------------
CONTROL.INPUT.ENC_INC2_COM_ANG = inc2_com_ang;
CONTROL.INPUT.ENC_INC2_DIF_ANG = inc2_dif_ang;
CONTROL.INPUT.ENC_INC_COM_ANG = inc_com_ang;
CONTROL.INPUT.ENC_INC_DIF_ANG = inc_dif_ang;
CONTROL.INPUT.ENC_DIF_ANG = dif_ang-dif_ang_offs;
CONTROL.INPUT.ENC_MOTOR_ANG = 2*pi/MOTOR_ENC_RES/MOTOR_GEAR_RATIO/WHEEL_GEAR_RATIO*[left_enc-left_enc_offs right_enc-right_enc_offs]';

return

== matlab function CAR_CONTROL_SYSTEM/GAZEBO SIMULATION/TCP_BRIDGE/TCP//IP SIM HW/YAW_ANGLE_DISTANCE_COMPUTATION ==
  data: LATERAL_DIST input; CONTROL output Bus: CONTROL_Bus; CONTROL_IN input
function CONTROL = WALL_ORIENTATION(LATERAL_DIST,CONTROL_IN)

%% UPDATE BUS
CONTROL = CONTROL_IN;
FRONT_DISTANCE = LATERAL_DIST(1);
REAR_DISTANCE = LATERAL_DIST(2);
%% PARAMETERS
RANGE_SENS_DIST = CONTROL.PARAM.RANGE_SENS_DIST;
%% MEASUREMENTS
CONTROL.INPUT.RANGE_WALL_ANG = atan2((REAR_DISTANCE-FRONT_DISTANCE),RANGE_SENS_DIST);
CONTROL.INPUT.RANGE_WALL_DIST = (FRONT_DISTANCE+REAR_DISTANCE)/2*cos(CONTROL.INPUT.RANGE_WALL_ANG);
CONTROL.INPUT.RANGE_FRONT_DIST = FRONT_DISTANCE; % m
CONTROL.INPUT.RANGE_REAR_DIST = REAR_DISTANCE; % m

return

== matlab function CAR_CONTROL_SYSTEM/HARDWARE/COMMUNICATIONS/TCP//IP RPI4/RPI4 CODER ==
  data: CONTROL input; TX_MSG output uint8
function TX_MSG  = RPI4_CODER(CONTROL)
%%%%%%%%%%%%%%%%%%%%%%%%%%%%%%%%%%%%%%%%%%%%%%%%%%%%%%%%%%%%%%%%%%%%%%%%%%%
% MCS MESSAGES
%%%%%%%%%%%%%%%%%%%%%%%%%%%%%%%%%%%%%%%%%%%%%%%%%%%%%%%%%%%%%%%%%%%%%%%%%%%
% WRITE IN THE CONTROL BUS
% RPi3 --> RPi4 (coder)
%       Odometría(48B): 3 single linear vel XYZ, 3 single ang vel RPY, 3 single posición XYZ y 3 single orientación XYZ.
%       GPS (24B): 3 double (float64) latitud, longitud, altitud
%       Estado (1B): 1 uint8
%       Tensión batería (4B): 1 single (float32)
%       Lidar ON (1B): 1 bool (uint8)
%             Total: 78B
TX_MSG = zeros(78,1,'uint8');
ii = 4*1; jj = 4;
TX_MSG(ii-jj+1:ii) = typecast(single(CONTROL.INPUT.FORWARD_VEL),'uint8');
% ii = 4*2; 
% TX_MSG(ii-jj+1:ii) = typecast(single(-CONTROL.INPUT.EARTH_VEL(2)),'uint8');
% ii = 4*3; 
% TX_MSG(ii-jj+1:ii) = typecast(single(-CONTROL.INPUT.EARTH_VEL(3)),'uint8');
ii = 4*6;
TX_MSG(ii-jj+1:ii) = typecast(single(-CONTROL.INPUT.YAW_RATE),'uint8');
if CONTROL.STATE.CONTROL_MODE == 2 || CONTROL.STATE.CONTROL_MODE == 3 ...
        || CONTROL.STATE.CONTROL_MODE == 6
    ii = 4*7;
    TX_MSG(ii-jj+1:ii) = typecast(single(CONTROL.INPUT.NAV_EARTH_POS_KF(1)),'uint8');
    ii = 4*8;
    TX_MSG(ii-jj+1:ii) = typecast(single(-CONTROL.INPUT.NAV_EARTH_POS_KF(2)),'uint8');
    % ii = 4*9;
    % TX_MSG(ii-jj+1:ii) = typecast(single(-CONTROL.INPUT.EARTH_POS(3)),'uint8');
    % ii = 4*10;
    % TX_MSG(ii-jj+1:ii) = typecast(single(CONTROL.INPUT.NAV_EULER_ANG(1)),'uint8');
    % ii = 4*11;
    % TX_MSG(ii-jj+1:ii) = typecast(single(-CONTROL.INPUT.NAV_EULER_ANG(2)),'uint8');
    ii = 4*12;
    TX_MSG(ii-jj+1:ii) = typecast(single(-CONTROL.INPUT.NAV_EULER_ANG_KF(3)),'uint8');
else
    ii = 4*7;
    TX_MSG(ii-jj+1:ii) = typecast(single(CONTROL.INPUT.MCS_EARTH_POS(1)),'uint8');
    ii = 4*8;
    TX_MSG(ii-jj+1:ii) = typecast(single(CONTROL.INPUT.MCS_EARTH_POS(2)),'uint8');
    ii = 4*9;
    TX_MSG(ii-jj+1:ii) = typecast(single(CONTROL.INPUT.MCS_EARTH_POS(3)),'uint8');
    ii = 4*10;
    TX_MSG(ii-jj+1:ii) = typecast(single(CONTROL.INPUT.MCS_EULER_ANG(1)),'uint8');
    ii = 4*11;
    TX_MSG(ii-jj+1:ii) = typecast(single(CONTROL.INPUT.MCS_EULER_ANG(2)),'uint8');
    ii = 4*12;
    TX_MSG(ii-jj+1:ii) = typecast(single(CONTROL.INPUT.MCS_EULER_ANG(3)),'uint8');
end
ii = 4*12 + 8*3 + 1; jj = 1;
TX_MSG(ii-jj+1:ii) = uint8(CONTROL.STATE.CURRENT_STATUS_SYS);
ii = 4*13 + 8*3 + 1; jj = 4;
TX_MSG(ii-jj+1:ii) = typecast(single(CONTROL.INPUT.BATTERY_VOLT),'uint8');
ii = 4*13 + 8*3 + 2; jj = 1;
TX_MSG(ii-jj+1:ii) = uint8(CONTROL.STATE.LIDAR_2D_MODE);

%%%%%%%%%%%%%%%%%%%%%%%%%%%%%%%%%%%%%%%%%%%%%%%%%%%%%%%%%%%%%%%%%%%%%%%%%%%


return

== matlab function CAR_CONTROL_SYSTEM/HARDWARE/COMMUNICATIONS/TCP//IP RPI4/RPI4 DECODER ==
  data: CONTROL_IN input; RX_MSG input; CONTROL output Bus: CONTROL_Bus; STATUS input
function CONTROL  = RPI4_DECODER(CONTROL_IN,RX_MSG,STATUS)
% Initialization
CONTROL = CONTROL_IN;
%%%%%%%%%%%%%%%%%%%%%%%%%%%%%%%%%%%%%%%%%%%%%%%%%%%%%%%%%%%%%%%%%%%%%%%%%%%
% MCS MESSAGES
%%%%%%%%%%%%%%%%%%%%%%%%%%%%%%%%%%%%%%%%%%%%%%%%%%%%%%%%%%%%%%%%%%%%%%%%%%%
% RPi4 --> RPi3 (decoder)
%       Referencia velocidad (24B): 3 single (float32) XYZ y 3 single RPY
%       Referencia pose (24B): 3 single posición XYZ y 3 single orientación XYZ
%       Pose real (24B): 3 single posición XYZ y 3 single orientación XYZ
%       GPS (24B): 3 double (float64) latitud, longitud, altitud
%       Botones (3B): 3 bool (uint8) A, B, C
%       Estado (1B): 1 byte (uint8)
%       Corriente de carga (4B): 1 single (float32)
%       Puntos lidar (480B): 120 single (ángulo 1.5º - 358.5º)
%       TOTAL: 584B
% WRITE IN THE CONTROL BUS
if STATUS==1
    %% FORWARD AND ANGULAR VELOCITY REFERENCES
    jj = 4;
    if CONTROL.STATE.CONTROL_MODE==1 || CONTROL.STATE.CONTROL_MODE==2
        ii = 4; 
        CONTROL.TARGET.FORWARD_VEL_REF_PC = double(typecast(RX_MSG(ii-jj+1:ii),'single'));
    end
    if CONTROL.STATE.CONTROL_MODE==2
        ii = 6*4;
        CONTROL.TARGET.YAW_RATE_REF_PC = double(-typecast(RX_MSG(ii-jj+1:ii),'single'));
    end
    %% POSE FROM RPI4
    if CONTROL.STATE.NAV_MODE>2
        ii = 13*4;
        CONTROL.INPUT.NAV_EARTH_POS(1) = double(typecast(RX_MSG(ii-jj+1:ii),'single'));
        ii = 14*4;
        CONTROL.INPUT.NAV_EARTH_POS(2) = double(-typecast(RX_MSG(ii-jj+1:ii),'single'));
        ii = 18*4;
        CONTROL.INPUT.NAV_EULER_ANG(3) = double(-typecast(RX_MSG(ii-jj+1:ii),'single'));
        % CONTROL.INPUT.YAW_ANG = double(-typecast(RX_MSG(ii-jj+1:ii),'single'));
    end
    %% POSE REFERENCES
    if CONTROL.STATE.NAV_TARGET_SOURCE == uint8(1) % PC
        ii = 7*4; jj = 4;
        CONTROL.TARGET.NAV_REF_PC(1) = double(typecast(RX_MSG(ii-jj+1:ii),'single'));
        ii = 8*4;
        CONTROL.TARGET.NAV_REF_PC(2) = double(-typecast(RX_MSG(ii-jj+1:ii),'single'));

    %%%%%%%%%  BUSSES FOR ANGLE AND POSITION NAVIGATION  %%%%%%%%%
    elseif CONTROL.STATE.NAV_TARGET_SOURCE == uint8(5) % EXTERNAL MISSION
        % MISSION_NUM_WAYPOINTS?
        CONTROL.PARAM.MISSION_COUNT = uint8(1);
        ii = 7*4; jj = 4;
        CONTROL.PARAM.MISSION_WAYPOINTS(1,2) = double(typecast(RX_MSG(ii-jj+1:ii),'single'));
        ii = 8*4;
        CONTROL.PARAM.MISSION_WAYPOINTS(1,3) = double(-typecast(RX_MSG(ii-jj+1:ii),'single'));
        ii = 12*4;
        CONTROL.PARAM.MISSION_WAYPOINTS(1,4) = double(-typecast(RX_MSG(ii-jj+1:ii),'single'));
        CONTROL.PARAM.MISSION_WAYPOINTS(1,1) = 1;
    end

    % if CONTROL.STATE.CONTROL_MODE==1
    %     ii = 12*4;
    %     CONTROL.TARGET.YAW_ANG_REF_PC = double(-typecast(RX_MSG(ii-jj+1:ii),'single'));
    % end

    %% UNWRAPPING
    yaw_ang_ref = CONTROL.TARGET.YAW_ANG_REF;
    yaw_ang = CONTROL.INPUT.NAV_EULER_ANG(3);
    angle_error = yaw_ang_ref - yaw_ang;
    if abs(angle_error) > pi
        if yaw_ang <= 0
            yaw_ang = yaw_ang + 2*pi;
        else
            yaw_ang = yaw_ang - 2*pi;
        end
        CONTROL.INPUT.NAV_EULER_ANG(3) = yaw_ang;
    end

    %% VIRTUAL BUTTONS
    ii = 18*4 + 3*8 + 1; jj = 1;
    CONTROL.STATE.NAV_BUTTONS(1) = RX_MSG(ii-jj+1:ii);
    ii = 18*4 + 3*8 + 2;
    CONTROL.STATE.NAV_BUTTONS(2) = RX_MSG(ii-jj+1:ii);
    ii = 18*4 + 3*8 + 3; 
    CONTROL.STATE.NAV_BUTTONS(3) = RX_MSG(ii-jj+1:ii);
    ii = 18*4 + 3*8 + 4;
    CONTROL.STATE.CURRENT_STATUS_RPI4 = RX_MSG(ii-jj+1:ii);
%     unused_local_variable = RX_MSG(ii-jj+1:ii);
    ii = 19*4 + 3*8 + 4; jj = 4;
    CONTROL.INPUT.CHARGING_CURRENT = double(typecast(RX_MSG(ii-jj+1:ii),'single'));
    for nn = 1:120
        CONTROL.INPUT.LIDAR_2D(nn,2) = double(typecast(RX_MSG(ii+4*nn-3:ii+4*nn),'single'));
    end
end
%%%%%%%%%%%%%%%%%%%%%%%%%%%%%%%%%%%%%%%%%%%%%%%%%%%%%%%%%%%%%%%%%%%%%%%%%%%


return
